simulink model "Schmitt_Trigger"  (R2024b)
settings: Solver=FixedStepAuto  StartTime=0.0  StopTime=20  FixedStep=0.01  RelTol=1e-3  EnableMultiTasking=on
libraries: stm32f4xxblockslib x1
settings Model: STM32="{\"AnalogInput\":[{\"ID\":\"BasicKit:1\"},{\"ID\":\"Potentiometer_Reader:1\"},{\"ID\":\"Schmitt_Trigger:14\"}],\"DigitalPortWrite\":{\"ID\":\"BasicKit:4\"},\"DigitalPortRead\":[{\"ID\":\"BasicKit:5\"},{\"ID\":\"BasicKit:7\"}]}"  Creator=pboon  LastModifiedBy=pboon
settings OptimizationCC: DefaultParameterBehavior=Inlined  EnhancedBackFolding=on  PassReuseOutputArgsAs=Individual arguments  ZeroExternalMemoryAtStartup=off  ZeroInternalMemoryAtStartup=off  MaxStackSize=512  OptimizeBlockOrder=speed  DifferentSizesBufferReuse=on  OptimizationCustomize=off  EfficientTunableParamExpr=on
settings DebuggingCC: ParameterTunabilityLossMsg=error
settings HardwareCC: ProdBitPerPointer=32  ProdBitPerSizeT=32  ProdBitPerPtrDiffT=32  ProdLargestAtomicInteger=Long  ProdLargestAtomicFloat=Double  ProdWordSize=32  ProdLongLongMode=on  ProdHWDeviceType=ARM Compatible->ARM Cortex-M
settings SFSimCC: MATLABDynamicMemAlloc=off
settings RTWCC: Description=Embedded Coder  SystemTargetFile=ert.tlc  HardwareBoard=STM32G4xx Based  TemplateMakefile=ert_default_tmf  Toolchain=GNU Tools for ARM Embedded Processors
settings CodeAppCC: ForceParamTrailComments=on  IgnoreCustomStorageClasses=off  OperatorAnnotations=on  SimulinkDataObjDesc=on  SFDataObjDesc=on  InsertBlockDesc=on
settings ERTTargetCC: TargetLangStandard=C99 (ISO)  CodeReplacementLibrary=ARM Cortex-M  ExtModeTransport=3  ExtModeStaticAlloc=on  ExtModeStaticAllocSize=2048  ExtModeMexFile=ext_xcp  ExtModeIntrfLevel=Level2 - Open

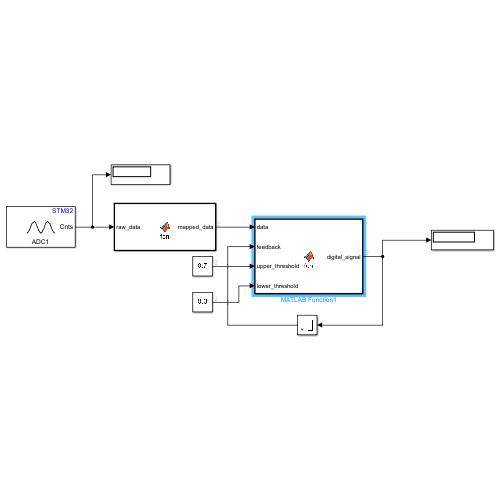
[thumbnail: Simulink's stored preview of the top-level diagram]
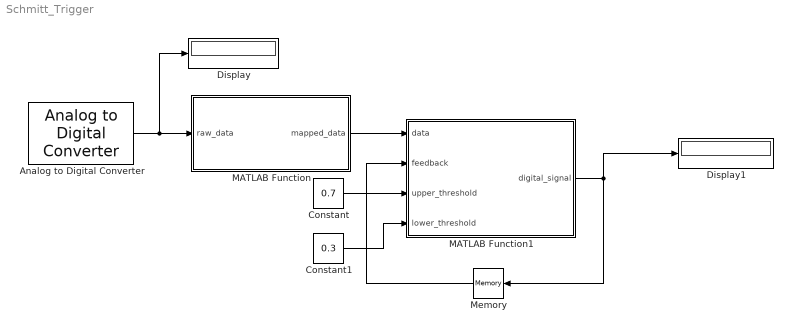
== system Schmitt_Trigger ==
  Analog to Digital Converter : stm32f4xxblockslib/Analog to Digital Converter  ADCModule=ADC1  ConversionGroup=Regular  TriggerMode=Trigger and read  NumberOfConversions=1  EnableBufferConv=off  BufferLength=1  OutputStatus=off  SampleTime=-1  EnableSimPort=off  hoistedMaskSrc=ECSoC/ECSimCodegen/Analog to Digital Converter
  Constant : Constant  Value=0.7
  Constant1 : Constant  Value=0.3
  Display : Display
  Display1 : Display
      settings: Format=bank
  MATLAB Function : MATLAB Function  TreatAsAtomicUnit=on
  MATLAB Function1 : MATLAB Function  TreatAsAtomicUnit=on
  Memory : Memory
  wires:
  Analog to Digital Converter/1 -> Display/1, MATLAB Function/1(raw_data)
  MATLAB Function/1(mapped_data) -> MATLAB Function1/1(data)
  MATLAB Function1/1(digital_signal) -> Memory/1, Display1/1
  Memory/1 -> MATLAB Function1/2(feedback)
  Constant/1 -> MATLAB Function1/3(upper_threshold)
  Constant1/1 -> MATLAB Function1/4(lower_threshold)

== matlab function Schmitt_Trigger/MATLAB Function1 ==
  data: data input; digital_signal output; feedback input; upper_threshold input; lower_threshold input
function digital_signal = fcn(data, feedback, upper_threshold, lower_threshold)
if data >= upper_threshold
    digital_signal = 1;
elseif data <= lower_threshold
    digital_signal = 0;
else
    digital_signal = feedback;
end

== matlab function Schmitt_Trigger/MATLAB Function ==
  data: raw_data input; mapped_data output
function mapped_data = fcn(raw_data)

in_min = 0.0;
out_min = 0.0;
in_max = 4095.0;
out_max = 1.0;

mapped_data =  (double(raw_data) - in_min) * (out_max - out_min) / (in_max - in_min) + out_min;
